simulink model "EPA_Jumper"  (R2018a)
settings: Solver=FixedStepDiscrete  StartTime=0.0  StopTime=inf  FixedStep=0.001  RelTol=1e-3  EnableMultiTasking=on
model workspace (MAT data in the model file):
  k_p_pam = Simulink.Parameter
  k_p_pam.DataType = 'auto'
  k_p_pam.Dimensions = [0 0]
values from neighbouring files (symbols this model uses):
  bits_current = 12    [Init_EPA_Jumper.m]
  bits_Kd = 12    [Init_EPA_Jumper.m]
  bits_Kp = 12    [Init_EPA_Jumper.m]
  bits_position = 16    [Init_EPA_Jumper.m]
  bits_velocity = 12    [Init_EPA_Jumper.m]
  KD_MAX = 5.0    (= 5)    [Init_EPA_Jumper.m]
  KD_MIN = 0.0    (= 0)    [Init_EPA_Jumper.m]
  KP_MAX = 500.0    (= 500)    [Init_EPA_Jumper.m]
  KP_MIN = 0.0    (= 0)    [Init_EPA_Jumper.m]
  P_MAX = 95.5    [Init_EPA_Jumper.m]
  P_MIN = -95.5    [Init_EPA_Jumper.m]
  PressureFilter_CutOffFreq = 20    [Init_EPA_Jumper.m]
  PressureFilter_Gain = 1    [Init_EPA_Jumper.m]
  ReadingVoltage = 5    [Init_EPA_Jumper.m]
  T_MAX = 18.0    (= 18)    [Init_EPA_Jumper.m]
  T_MIN = -18.0    (= -18)    [Init_EPA_Jumper.m]
  V_MAX = 45.0    (= 45)    [Init_EPA_Jumper.m]
  V_MIN = -45.0    (= -45)    [Init_EPA_Jumper.m]
  voltageBias = -2.5    [Init_EPA_Jumper.m]
  voltageMultiplier = 2.5    [Init_EPA_Jumper.m]
  VoltageResolution = 1023.0    (= 1023)    [Init_EPA_Jumper.m]
libraries: xpcethercatlib x76, slrtlib x15, simulink x10, peGeneralControl x9
(part 1 of 3)
settings Model: xpc_rtwmakecfg_data=_xpcethercatlib_  SimulationMode=external  Creator=marcm  LastModifiedBy=Lauflabor
settings SolverCC: ConcurrentTasks=on  AutoInsertRateTranBlk=on
settings DataIOCC: SaveFormat=StructureWithTime
settings OptimizationCC: BlockReduction=off  OptimizeBlockIOStorage=off  BufferReuse=off  GlobalBufferReuse=off  ExpressionFolding=off  LocalBlockOutputs=off  OptimizeDataStoreBuffers=off  BusAssignmentInplaceUpdate=off
settings HardwareCC: ProdBitPerPointer=32  ProdBitPerSizeT=32  ProdBitPerPtrDiffT=32  ProdLargestAtomicFloat=None  ProdWordSize=32  ProdLongLongMode=on  ProdHWDeviceType=Generic->32-bit x86 compatible
settings RTWCC: SystemTargetFile=slrt.tlc  TemplateMakefile=slrt_default_tmf  Description=Simulink Real-Time  CodeExecutionProfiling=on  RTWCompilerOptimization=on
settings CodeAppCC: StateflowObjectComments=on
settings SimulinkRealTimeCC: SupportVariableSizeSignals=on  xPCConcurrentTasks=on

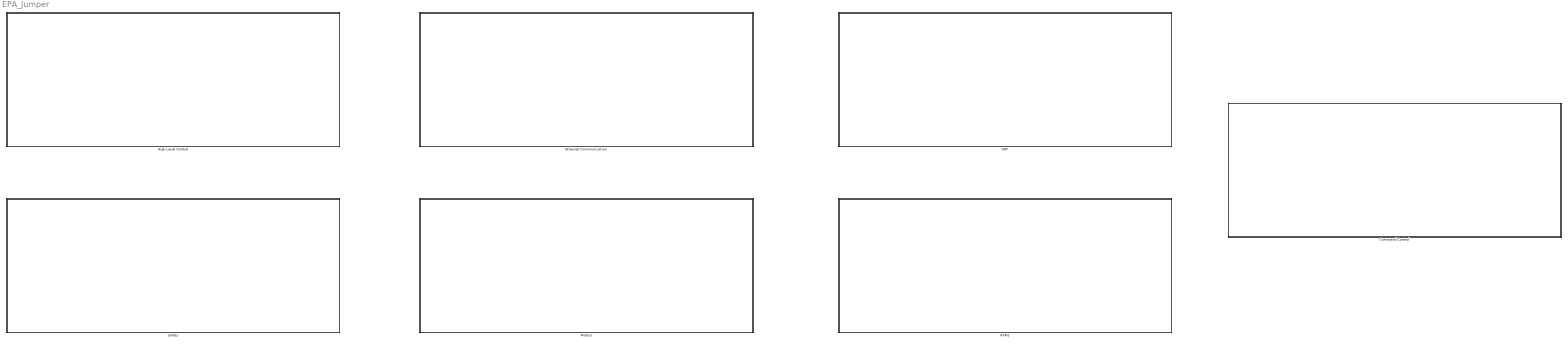
== system EPA_Jumper ==
  Command Control : Subsystem
  Ethernet Communication : Subsystem
  GRF : Subsystem
  High Level Control : Subsystem
  Motors : Subsystem
  PAMs : Subsystem
  "Safety " : Subsystem

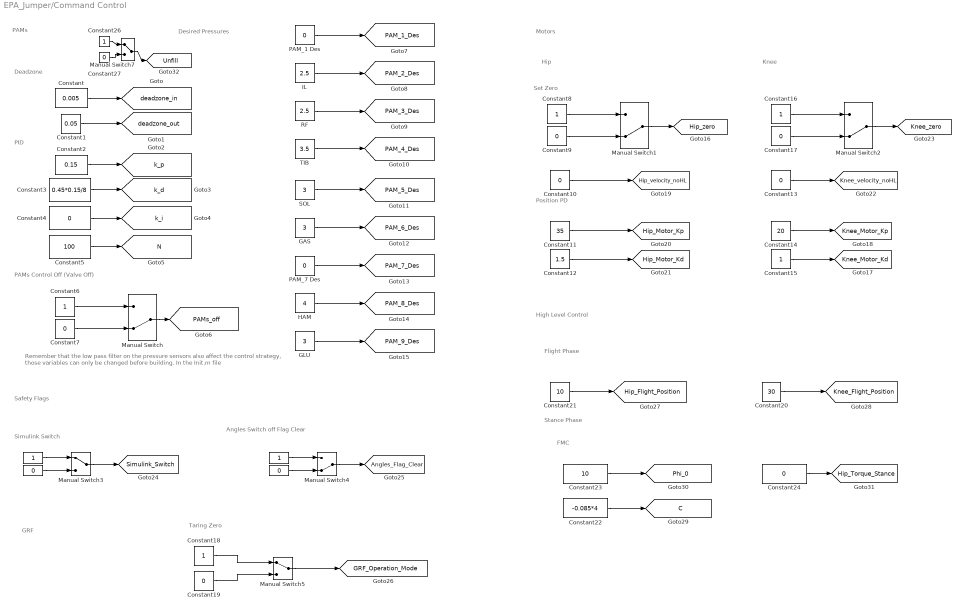
== system EPA_Jumper/Command Control ==
  note: PID
  note: PAMs
  note: Deadzone
  note: PAMs Control Off (Valve Off)
  note: Desired Pressures
  note: Motors
  note: Remember that the low pass filter on the pressure sensors also affect the control strategy, those variables can only be changed before building. In the Init.m file
  note: Hip
  note: Knee
  note: Safety Flags
  note: Simulink Switch
  note: Angles Switch off Flag Clear
  note: Taring Zero
  note: GRF
  note: High Level Control
  note: Flight Phase
  note: Stance Phase
  note: FMC
  note: Position PD
  note: Set Zero
  " " : Constant
  "   " : Constant  Value=0
  "    " : Constant  Value=0
  "               " : Constant
  Constant : Constant  Value=0.005
  Constant1 : Constant  Value=0.05
  Constant{4,7,9..10,13,17,19,24,27} (9 alike) : Constant  Value=0
  Constant11 : Constant  Value=35
  Constant12 : Constant  Value=1.5
  Constant14 : Constant  Value=20
  Constant{6,8,15..16,18,26} (6 alike) : Constant
  Constant2 : Constant  Value=0.15
  Constant20 : Constant  Value=30
  Constant21 : Constant  Value=10
  Constant22 : Constant  Value=-0.085*4
  Constant23 : Constant  Value=10
  Constant3 : Constant  Value=0.45*0.15/8
  Constant5 : Constant  Value=100
  GAS : Constant  Value=3
  GLU : Constant  Value=3
  HAM : Constant  Value=4
  IL : Constant  Value=2.5
  Manual Switch{,1..2,4} (4 alike) : ManualSwitch  CurrentSetting=0
  Manual Switch3 : ManualSwitch
  Manual Switch5 : ManualSwitch
  Manual Switch7 : ManualSwitch
  PAM_1 Des : Constant  Value=0
  PAM_7 Des : Constant  Value=0
  RF : Constant  Value=2.5
  SOL : Constant  Value=3
  TIB : Constant  Value=3.5
  tag scope: Angles_Flag_Clear=global, C=global, GRF_Operation_Mode=global, Hip_Flight_Position=global, Hip_Motor_Kd=global, Hip_Motor_Kp=global, Hip_Torque_Stance=global, Hip_velocity_noHL=global, Hip_zero=global, Knee_Flight_Position=global, Knee_Motor_Kd=global, Knee_Motor_Kp=global, Knee_velocity_noHL=global, Knee_zero=global, N=global, PAM_1_Des=global, PAM_2_Des=global, PAM_3_Des=global, PAM_4_Des=global, PAM_5_Des=global, PAM_6_Des=global, PAM_7_Des=global, PAM_8_Des=global, PAM_9_Des=global, PAMs_off=global, Phi_0=global, Simulink_Switch=global, Unfill=global, deadzone_in=global, deadzone_out=global, k_d=global, k_i=global, k_p=global
  wires:
  Constant5/1 -> [N]
  Constant4/1 -> [k_i]
  Constant6/1 -> Manual Switch/1
  Manual Switch/1 -> [PAMs_off]
  Constant1/1 -> [deadzone_out]
  Constant7/1 -> Manual Switch/2
  Constant2/1 -> [k_p]
  Constant/1 -> [deadzone_in]
  Constant3/1 -> [k_d]
  PAM_1 Des/1 -> [PAM_1_Des]
  IL/1 -> [PAM_2_Des]
  RF/1 -> [PAM_3_Des]
  TIB/1 -> [PAM_4_Des]
  SOL/1 -> [PAM_5_Des]
  GAS/1 -> [PAM_6_Des]
  PAM_7 Des/1 -> [PAM_7_Des]
  HAM/1 -> [PAM_8_Des]
  GLU/1 -> [PAM_9_Des]
  Constant8/1 -> Manual Switch1/1
  Constant9/1 -> Manual Switch1/2
  Manual Switch1/1 -> [Hip_zero]
  Constant10/1 -> [Hip_velocity_noHL]
  Constant11/1 -> [Hip_Motor_Kp]
  Constant12/1 -> [Hip_Motor_Kd]
  Constant13/1 -> [Knee_velocity_noHL]
  Constant14/1 -> [Knee_Motor_Kp]
  Constant15/1 -> [Knee_Motor_Kd]
  Manual Switch2/1 -> [Knee_zero]
  Constant17/1 -> Manual Switch2/2
  Constant16/1 -> Manual Switch2/1
  " "/1 -> Manual Switch3/1
  "    "/1 -> Manual Switch3/2
  Manual Switch3/1 -> [Simulink_Switch]
  Manual Switch4/1 -> [Angles_Flag_Clear]
  "               "/1 -> Manual Switch4/1
  "   "/1 -> Manual Switch4/2
  Manual Switch5/1 -> [GRF_Operation_Mode]
  Constant18/1 -> Manual Switch5/1
  Constant19/1 -> Manual Switch5/2
  Constant21/1 -> [Hip_Flight_Position]
  Constant20/1 -> [Knee_Flight_Position]
  Constant23/1 -> [Phi_0]
  Constant22/1 -> [C]
  Constant24/1 -> [Hip_Torque_Stance]
  Constant26/1 -> Manual Switch7/1
  Constant27/1 -> Manual Switch7/2
  Manual Switch7/1 -> [Unfill]

== system EPA_Jumper/Ethernet Communication ==
  "EtherCAT Get Notifications " : xpcethercatlib/EtherCAT Get Notifications   device_id=0  sample_time=.001
      settings: SourceProductName=Simulink Real-Time  SourceProductBaseCode=XP
  "EtherCAT Init " : xpcethercatlib/EtherCAT Init   Priority=0  config_file=C:\Users\Lauflabor\Documents\EPA Jumper\RealTime Code\EPA_Jumper_2.xml  device_id=0  pci_bus=1  pci_slot=0  pci_function=0  dctuning=0  enaDebug=on  enaDC=on  errLink=off  masterDbg=on  stateChgDbg=on  baseClock=on  masterCfg=off  logFile='c:\dbglog.txt'  sample_time=0.001000  DCMode=0
      settings: SourceProductName=Simulink Real-Time  SourceProductBaseCode=XP
  Inputs : Subsystem
  Outputs : Subsystem
  Terminator : Terminator
  Terminator1 : Terminator
  wires:
  "EtherCAT Get Notifications "/1 -> Terminator1/1
  "EtherCAT Init "/1 -> Terminator/1

== system EPA_Jumper/GRF ==
  note: GRF Meassures
  GRFx : Subsystem
  GRFy : Subsystem
  GRFz : Subsystem

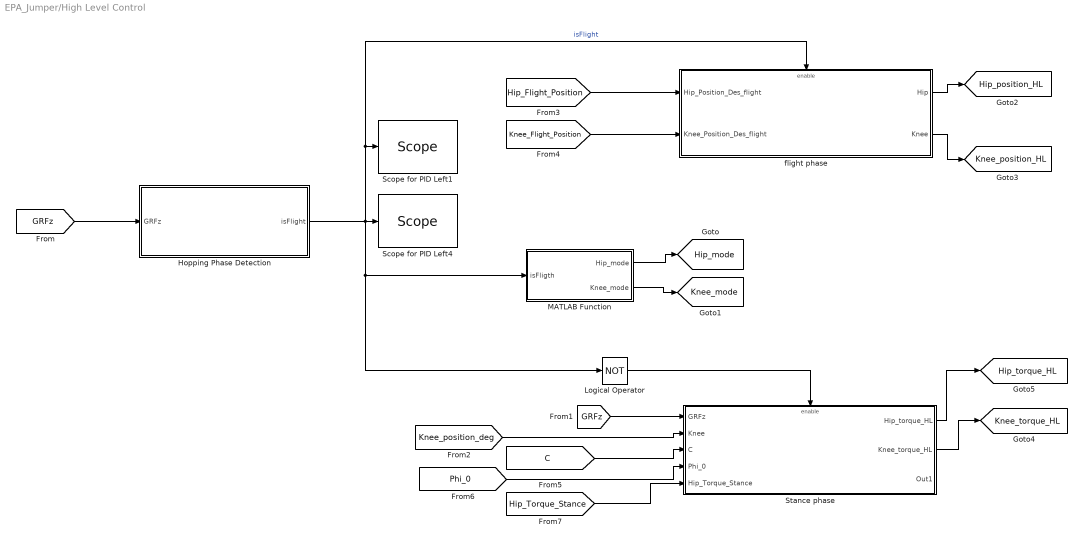
== system EPA_Jumper/High Level Control ==
  Hopping Phase Detection : MATLAB Function  TreatAsAtomicUnit=on
  Logical Operator : Logic  Operator=NOT  AllPortsSameDT=off  OutDataTypeStr=boolean
  MATLAB Function : MATLAB Function  TreatAsAtomicUnit=on
  Scope for PID Left1 : slrtlib/Displays and Logging/Scope   scopeno=7  scopetype=File  autostart=on  viewmode=Graphical sliding  formatstr='%15.6f'  grid=on  ylimits=[-0.5, 1.5]  nosamples=1000000  noprepostsamples=0  interleave=1  triggermode=FreeRun  triggersignal=1  trigsignalfromport=off  triggerlevel=0.0  triggerslope=Either  triggerscope=1  triggersample=0  filename=isFlight.dat  mode=Lazy  writesize=512  autorestart=off  dynamicfilemode=off  maxwritefilesize=512*1024^2
  Scope for PID Left4 : slrtlib/Displays and Logging/Scope   scopeno=6  scopetype=Target  autostart=on  viewmode=Graphical sliding  formatstr='%15.6f'  grid=on  ylimits=[-0.5, 1.5]  nosamples=1000  noprepostsamples=0  interleave=1  triggermode=FreeRun  triggersignal=1  trigsignalfromport=off  triggerlevel=0.0  triggerslope=Either  triggerscope=1  triggersample=0  filename=data.dat  mode=Lazy  writesize=512  autorestart=off  dynamicfilemode=off  maxwritefilesize=512*1024^2
  Stance phase : Subsystem
  flight phase : Subsystem
  tag scope: Hip_mode=global, Hip_position_HL=global, Hip_torque_HL=global, Knee_mode=global, Knee_position_HL=global, Knee_torque_HL=global
  wires:
  Hopping Phase Detection/1(isFlight) -> Scope for PID Left1/1, flight phase/Enable, Scope for PID Left4/1, MATLAB Function/1(isFligth), Logical Operator/1  "isFlight"
  [GRFz] -> Hopping Phase Detection/1(GRFz)
  [Hip_Flight_Position] -> flight phase/1(Hip_Position_Des_flight)
  [Knee_Flight_Position] -> flight phase/2(Knee_Position_Des_flight)
  Logical Operator/1 -> Stance phase/Enable
  MATLAB Function/1(Hip_mode) -> [Hip_mode]
  MATLAB Function/2(Knee_mode) -> [Knee_mode]
  flight phase/1(Hip) -> [Hip_position_HL]
  flight phase/2(Knee) -> [Knee_position_HL]
  [GRFz] -> Stance phase/1("GRFz ")
  [Knee_position_deg] -> Stance phase/2(Knee)
  Stance phase/2(Knee_torque_HL) -> [Knee_torque_HL]
  Stance phase/1(Hip_torque_HL) -> [Hip_torque_HL]
  [C] -> Stance phase/3(C)
  [Phi_0] -> Stance phase/4(Phi_0)
  [Hip_Torque_Stance] -> Stance phase/5(Hip_Torque_Stance)

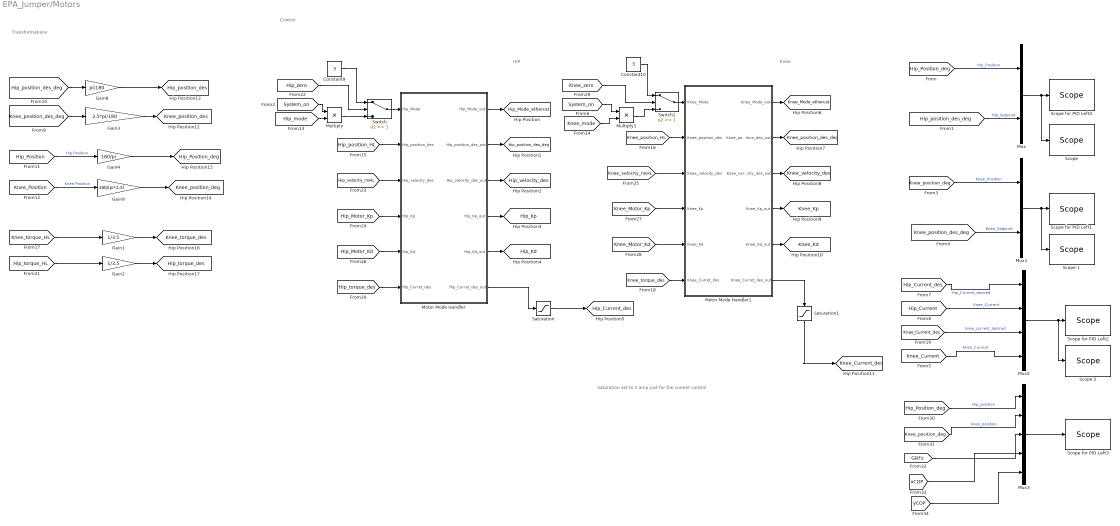
== system EPA_Jumper/Motors ==
  note: Saturation set to 5 amp just for the current control
  note: HIP
  note: Knee
  note: Control
  note: Transformations
  Constant10 : Constant  Value=3
  Constant9 : Constant  Value=3
  Gain1 : Gain  Gain=1/3.5
  Gain2 : Gain  Gain=1/3.5
  Gain3 : Gain  Gain=2.5*pi/180
  Gain4 : Gain  Gain=180/pi
  Gain8 : Gain  Gain=pi/180
  Gain9 : Gain  Gain=180/(pi*2.5)
  Motor Mode Handler : MATLAB Function  TreatAsAtomicUnit=on
  Motor Mode Handler1 : MATLAB Function  TreatAsAtomicUnit=on
  Multiply : Product
  Multiply1 : Product
  Mux : Mux  Inputs=2
  Mux1 : Mux  Inputs=2
  Mux2 : Mux
  Mux3 : Mux  Inputs=5
  Saturation : Saturate  UpperLimit=10  LowerLimit=-10
  Saturation1 : Saturate  UpperLimit=10  LowerLimit=-10
  "Scope " : slrtlib/Displays and Logging/Scope   scopeno=12  scopetype=File  autostart=on  viewmode=Graphical redraw  formatstr='%15.6f'  grid=on  ylimits=[0,0]  nosamples=1000000  noprepostsamples=0  interleave=1  triggermode=FreeRun  triggersignal=1  trigsignalfromport=off  triggerlevel=0.0  triggerslope=Either  triggerscope=1  triggersample=0  filename=hipPos.dat  mode=Lazy  writesize=512  autorestart=off  dynamicfilemode=off  maxwritefilesize=512*1024^2
  Scope 1 : slrtlib/Displays and Logging/Scope   scopeno=13  scopetype=File  autostart=on  viewmode=Graphical redraw  formatstr='%15.6f'  grid=on  ylimits=[0,0]  nosamples=1000000  noprepostsamples=0  interleave=1  triggermode=FreeRun  triggersignal=1  trigsignalfromport=off  triggerlevel=0.0  triggerslope=Either  triggerscope=1  triggersample=0  filename=kneePos.dat  mode=Lazy  writesize=512  autorestart=off  dynamicfilemode=off  maxwritefilesize=512*1024^2
  Scope 2 : slrtlib/Displays and Logging/Scope   scopeno=14  scopetype=File  autostart=on  viewmode=Graphical redraw  formatstr='%15.6f'  grid=on  ylimits=[0,0]  nosamples=1000000  noprepostsamples=0  interleave=1  triggermode=FreeRun  triggersignal=1  trigsignalfromport=off  triggerlevel=0.0  triggerslope=Either  triggerscope=1  triggersample=0  filename=motCurr.dat  mode=Lazy  writesize=512  autorestart=off  dynamicfilemode=off  maxwritefilesize=512*1024^2
  Scope for PID Left1 : slrtlib/Displays and Logging/Scope   scopeno=4  scopetype=Target  autostart=on  viewmode=Graphical sliding  formatstr='%15.6f'  grid=on  ylimits=[-10, 120]  nosamples=1000  noprepostsamples=0  interleave=1  triggermode=FreeRun  triggersignal=1  trigsignalfromport=off  triggerlevel=0.0  triggerslope=Either  triggerscope=1  triggersample=0  filename=data.dat  mode=Lazy  writesize=512  autorestart=off  dynamicfilemode=off  maxwritefilesize=512*1024^2
  Scope for PID Left2 : slrtlib/Displays and Logging/Scope   scopeno=5  scopetype=Target  autostart=on  viewmode=Numerical  formatstr='%15.6f'  grid=on  ylimits=[0, 0]  nosamples=1000  noprepostsamples=0  interleave=1  triggermode=FreeRun  triggersignal=1  trigsignalfromport=off  triggerlevel=0.0  triggerslope=Either  triggerscope=1  triggersample=0  filename=data.dat  mode=Lazy  writesize=512  autorestart=off  dynamicfilemode=off  maxwritefilesize=512*1024^2
  Scope for PID Left3 : slrtlib/Displays and Logging/Scope   scopeno=9  scopetype=Target  autostart=on  viewmode=Numerical  formatstr='%15.6f'  grid=on  ylimits=[0, 0]  nosamples=500  noprepostsamples=0  interleave=1  triggermode=FreeRun  triggersignal=1  trigsignalfromport=off  triggerlevel=0.0  triggerslope=Either  triggerscope=1  triggersample=0  filename=data.dat  mode=Lazy  writesize=512  autorestart=off  dynamicfilemode=off  maxwritefilesize=512*1024^2
  Scope for PID Left4 : slrtlib/Displays and Logging/Scope   scopeno=3  scopetype=Target  autostart=on  viewmode=Graphical sliding  formatstr='%15.6f'  grid=on  ylimits=[-60, 60]  nosamples=1000  noprepostsamples=0  interleave=1  triggermode=FreeRun  triggersignal=1  trigsignalfromport=off  triggerlevel=0.0  triggerslope=Either  triggerscope=1  triggersample=0  filename=data.dat  mode=Lazy  writesize=512  autorestart=off  dynamicfilemode=off  maxwritefilesize=512*1024^2
  Switch : Switch  Threshold=1
  Switch1 : Switch  Threshold=1
  tag scope: Hip_Current_des=global, Hip_Kd=global, Hip_Kp=global, Hip_Mode_ethercat=global, Hip_Position_deg=global, Hip_position_des=global, Hip_position_des_deg=global, Hip_torque_des=global, Hip_velocity_des=global, Knee_Current_des=global, Knee_Kd=global, Knee_Kp=global, Knee_Mode_ethercat=global, Knee_position_deg=global, Knee_position_des=global, Knee_position_des_deg=global, Knee_torque_des=global, Knee_velocity_des=global
  wires:
  Motor Mode Handler/3(Hip_velocity_des_out) -> [Hip_velocity_des]
  Motor Mode Handler/4(Hip_Kp_out) -> [Hip_Kp]
  Motor Mode Handler/5(Hip_Kd_out) -> [Hip_Kd]
  Motor Mode Handler/6(Hip_Curret_des_out) -> Saturation/1
  Motor Mode Handler/2(Hip_position_des_out) -> [Hip_position_des_deg]
  [Hip_position_des_deg] -> Mux/2  "Hip_Setpoint"
  [Hip_Position_deg] -> Mux/1  "Hip_Position"
  Mux/1 -> "Scope "/1, Scope for PID Left4/1
  Mux1/1 -> Scope 1/1, Scope for PID Left1/1
  [Knee_position_des_deg] -> Mux1/2  "Knee_Setpoint"
  Mux2/1 -> Scope 2/1, Scope for PID Left2/1
  Multiply/1 -> Switch/3
  [System_on] -> Multiply/1
  Motor Mode Handler/1(Hip_Mode_out) -> [Hip_Mode_ethercat]
  [Hip_position_HL] -> Motor Mode Handler/2(Hip_position_des)
  [Hip_velocity_noHL] -> Motor Mode Handler/3(Hip_velocity_des)
  [Hip_Motor_Kp] -> Motor Mode Handler/4(Hip_Kp)
  [Hip_Motor_Kd] -> Motor Mode Handler/5(Hip_Kd)
  [Hip_torque_des] -> Motor Mode Handler/6(Hip_Curret_des)
  [Knee_position_HL] -> Motor Mode Handler1/2(Knee_position_des)
  [System_on] -> Multiply1/1
  Motor Mode Handler1/5(Knee_Kd_out) -> [Knee_Kd]
  Motor Mode Handler1/1(Knee_Mode_out) -> [Knee_Mode_ethercat]
  Motor Mode Handler1/2(Knee_position_des_out) -> [Knee_position_des_deg]
  Motor Mode Handler1/3(Knee_velocity_des_out) -> [Knee_velocity_des]
  Motor Mode Handler1/4(Knee_Kp_out) -> [Knee_Kp]
  Motor Mode Handler1/6(Knee_Curret_des_out) -> Saturation1/1
  [Knee_position_deg] -> Mux1/1  "Knee_Position"
  [Hip_position_des_deg] -> Gain8/1
  [Knee_position_des_deg] -> Gain3/1
  [Hip_Position] -> Gain4/1  "Hip Position"
  [Knee_Position] -> Gain9/1  "Knee Position"
  Gain3/1 -> [Knee_position_des]
  Gain8/1 -> [Hip_position_des]
  Gain9/1 -> [Knee_position_deg]
  Gain4/1 -> [Hip_Position_deg]
  [Knee_torque_HL] -> Gain1/1
  Gain1/1 -> [Knee_torque_des]
  [Hip_mode] -> Multiply/2
  Constant9/1 -> Switch/1
  [Knee_mode] -> Multiply1/2
  Constant10/1 -> Switch1/1
  Switch/1 -> Motor Mode Handler/1(Hip_Mode)
  Switch1/1 -> Motor Mode Handler1/1(Knee_Mode)
  [Knee_torque_des] -> Motor Mode Handler1/6(Knee_Curret_des)
  Saturation/1 -> [Hip_Current_des]
  Saturation1/1 -> [Knee_Current_des]
  [Hip_torque_HL] -> Gain2/1
  Gain2/1 -> [Hip_torque_des]
  [Hip_zero] -> Switch/2
  [Knee_velocity_noHL] -> Motor Mode Handler1/3(Knee_velocity_des)
  [Knee_Motor_Kp] -> Motor Mode Handler1/4(Knee_Kp)
  [Knee_Motor_Kd] -> Motor Mode Handler1/5(Knee_Kd)
  Multiply1/1 -> Switch1/3
  [Knee_zero] -> Switch1/2
  Mux3/1 -> Scope for PID Left3/1
  [Hip_Position_deg] -> Mux3/1  "Hip_position"
  [Knee_position_deg] -> Mux3/2  "knee_position"
  [Hip_Current_des] -> Mux2/1  "Hip_Current_desired"
  [Hip_Current] -> Mux2/2  "Knee_Current"
  [Knee_Current_des] -> Mux2/3  "knee_current_desired"
  [Knee_Current] -> Mux2/4  "Knee_Current"
  [GRFz] -> Mux3/3
  [xCOP] -> Mux3/4
  [yCOP] -> Mux3/5

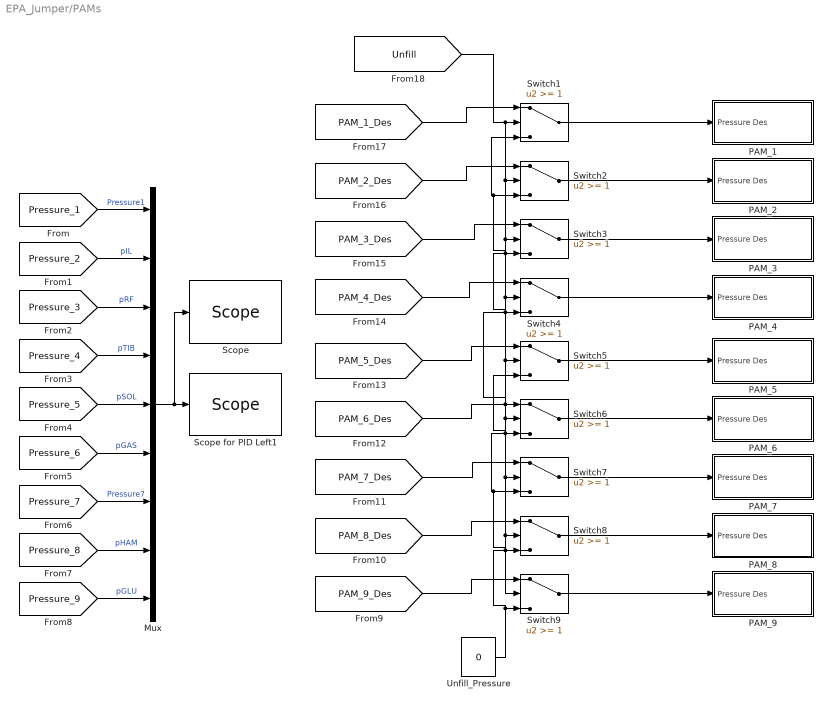
== system EPA_Jumper/PAMs ==
  Mux : Mux  Inputs=9
  PAM_1 : Subsystem
  PAM_2 : Subsystem
  PAM_3 : Subsystem
  PAM_4 : Subsystem
  PAM_5 : Subsystem
  PAM_6 : Subsystem
  PAM_7 : Subsystem
  PAM_8 : Subsystem
  PAM_9 : Subsystem
  "Scope " : slrtlib/Displays and Logging/Scope   scopeno=15  scopetype=File  autostart=on  viewmode=Graphical redraw  formatstr='%15.6f'  grid=on  ylimits=[0,0]  nosamples=1000000  noprepostsamples=0  interleave=1  triggermode=FreeRun  triggersignal=1  trigsignalfromport=off  triggerlevel=0.0  triggerslope=Either  triggerscope=1  triggersample=0  filename=pressure.dat  mode=Lazy  writesize=512  autorestart=off  dynamicfilemode=off  maxwritefilesize=512*1024^2
  Scope for PID Left1 : slrtlib/Displays and Logging/Scope   scopeno=8  scopetype=Target  autostart=on  viewmode=Numerical  formatstr='%15.6f'  grid=on  ylimits=[0, 120]  nosamples=1000  noprepostsamples=0  interleave=1  triggermode=FreeRun  triggersignal=1  trigsignalfromport=off  triggerlevel=0.0  triggerslope=Either  triggerscope=1  triggersample=0  filename=data.dat  mode=Lazy  writesize=512  autorestart=off  dynamicfilemode=off  maxwritefilesize=512*1024^2
  Switch{1..9} (9 alike) : Switch  Threshold=1
  Unfill_Pressure : Constant  Value=0
  wires:
  Mux/1 -> "Scope "/1, Scope for PID Left1/1
  [Pressure_1] -> Mux/1  "Pressure1"
  [Pressure_2] -> Mux/2  "pIL"
  [Pressure_3] -> Mux/3  "pRF"
  [Pressure_4] -> Mux/4  "pTIB"
  [Pressure_5] -> Mux/5  "pSOL"
  [Pressure_6] -> Mux/6  "pGAS"
  [Pressure_7] -> Mux/7  "Pressure7"
  [Pressure_8] -> Mux/8  "pHAM"
  [Pressure_9] -> Mux/9  "pGLU"
  [PAM_9_Des] -> Switch9/1
  Switch8/1 -> PAM_8/1(Pressure Des)
  Switch7/1 -> PAM_7/1(Pressure Des)
  [PAM_7_Des] -> Switch7/1
  [PAM_8_Des] -> Switch8/1
  [PAM_1_Des] -> Switch1/1
  Switch1/1 -> PAM_1/1(Pressure Des)
  [PAM_2_Des] -> Switch2/1
  Switch2/1 -> PAM_2/1(Pressure Des)
  [PAM_3_Des] -> Switch3/1
  Switch3/1 -> PAM_3/1(Pressure Des)
  [PAM_4_Des] -> Switch4/1
  Switch4/1 -> PAM_4/1(Pressure Des)
  [PAM_5_Des] -> Switch5/1
  Switch5/1 -> PAM_5/1(Pressure Des)
  Switch6/1 -> PAM_6/1(Pressure Des)
  [PAM_6_Des] -> Switch2/3, Switch1/3, Switch3/3, Switch4/3, Switch6/1
  [Unfill] -> Switch9/2, Switch8/2, Switch7/2, Switch6/2, Switch5/2, Switch4/2, Switch3/2, Switch2/2, Switch1/2
  Switch9/1 -> PAM_9/1(Pressure Des)
  Unfill_Pressure/1 -> Switch7/3, Switch5/3, Switch6/3, Switch8/3, Switch9/3

== system EPA_Jumper/Safety  ==
  AND1 : Logic  IconShape=distinctive  AllPortsSameDT=off  OutDataTypeStr=boolean
  Delay : Delay  DelayLength=1  InitialCondition=0  ExternalReset=Either
      settings: InputPortMap=u0,r5
  MATLAB Function : MATLAB Function  TreatAsAtomicUnit=on
  Mux : Mux  Inputs=6
  "Scope " : slrtlib/Displays and Logging/Scope   scopeno=11  scopetype=File  autostart=on  viewmode=Graphical redraw  formatstr='%15.6f'  grid=on  ylimits=[0,0]  nosamples=1000000  noprepostsamples=0  interleave=1  triggermode=FreeRun  triggersignal=1  trigsignalfromport=off  triggerlevel=0.0  triggerslope=Either  triggerscope=1  triggersample=0  filename=safety.dat  mode=Lazy  writesize=512  autorestart=off  dynamicfilemode=off  maxwritefilesize=512*1024^2
  Scope for PID Left4 : slrtlib/Displays and Logging/Scope   scopeno=2  scopetype=Target  autostart=on  viewmode=Numerical  formatstr='%15.6f'  grid=on  ylimits=[0, 0]  nosamples=1000  noprepostsamples=0  interleave=1  triggermode=FreeRun  triggersignal=1  trigsignalfromport=off  triggerlevel=0.0  triggerslope=Either  triggerscope=1  triggersample=0  filename=data.dat  mode=Lazy  writesize=512  autorestart=off  dynamicfilemode=off  maxwritefilesize=512*1024^2
  System On : Subsystem
  tag scope: System_on=global
  wires:
  System On/1(System On) -> Mux/1, AND1/1  "System_On"
  [Simulink_Switch] -> Mux/2, System On/1("Simulink Switch ")  "Simulink_wwitch"
  Mux/1 -> "Scope "/1, Scope for PID Left4/1
  System On/2(Emergency) -> Mux/3  "Emergency_switch"
  [Hip_Position_deg] -> MATLAB Function/1(Hip_Position)
  [Knee_position_deg] -> MATLAB Function/2(Knee_Position)
  MATLAB Function/3(Motors_safe) -> AND1/2, Mux/4  "Motors_safe"
  MATLAB Function/1(Hip_motor_safe) -> Mux/5  "Hip_motor_safe"
  MATLAB Function/2(Knee_motor_safe) -> Mux/6  "Knee_motor_safe"
  AND1/1 -> [System_on]  "System_On"
  MATLAB Function/4(flag) -> Delay/1
  Delay/1 -> MATLAB Function/3(flag_1)
  [Angles_Flag_Clear] -> Delay/2

== system EPA_Jumper/Ethernet Communication/Inputs ==
  GRF Slave : Subsystem
  Motor Slave : Subsystem
  PAMs Slave : Subsystem

== system EPA_Jumper/Ethernet Communication/Outputs ==
  GRF Slave : Subsystem
  Motor Slave : Subsystem
  PAMs Slave : Subsystem

== system EPA_Jumper/GRF/GRFx ==

== system EPA_Jumper/GRF/GRFy ==

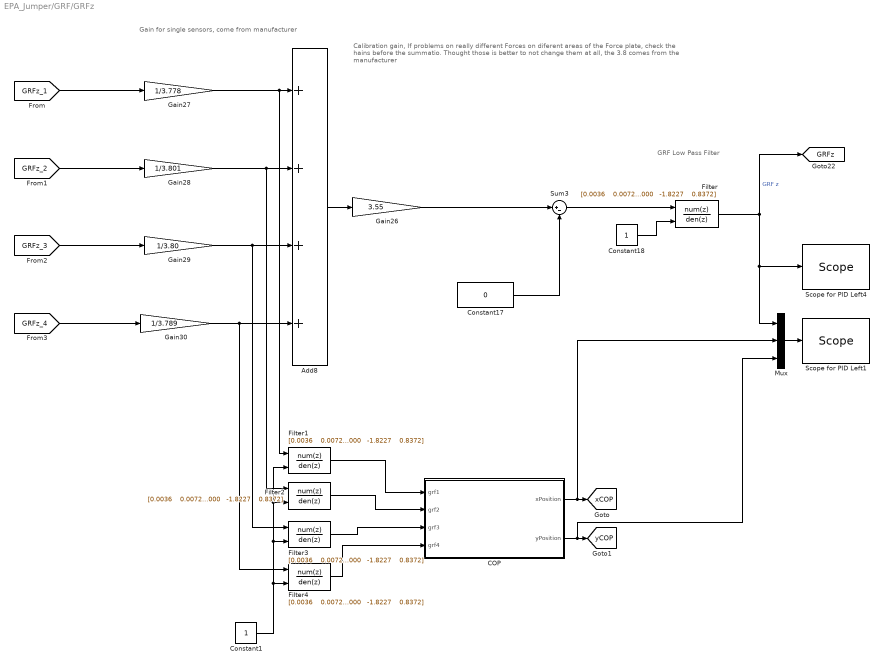
== system EPA_Jumper/GRF/GRFz ==
  note: Calibration gain, If problems on really different Forces on diferent areas of the Force plate, check the hains before the summatio. Thought those is better to not change them at all, the 3.8 comes from the manufacturer
  note: GRF Low Pass Filter
  note: Gain for single sensors, come from manufacturer
  Add8 : Sum  Inputs=++++
  COP : MATLAB Function  TreatAsAtomicUnit=on
  Constant1 : Constant
  Constant17 : Constant  Value=0
  Constant18 : Constant
  Filter{,1..4} (5 alike) : DiscreteFilter  Numerator="[0.0036    0.0072    0.0036]"  Denominator="[1.0000   -1.8227    0.8372]"  ExternalReset=Either
      settings: InputPortMap=u0,r7
  Gain26 : Gain  Gain=3.55
  Gain27 : Gain  Gain=1/3.778
  Gain28 : Gain  Gain=1/3.801
  Gain29 : Gain  Gain=1/3.80
  Gain30 : Gain  Gain=1/3.789
  Mux : Mux  Inputs=3
  Scope for PID Left1 : slrtlib/Displays and Logging/Scope   scopeno=10  scopetype=File  autostart=on  viewmode=Graphical sliding  formatstr='%15.6f'  grid=on  ylimits=[0, 100]  nosamples=1000000  noprepostsamples=0  interleave=1  triggermode=FreeRun  triggersignal=1  trigsignalfromport=off  triggerlevel=0.0  triggerslope=Either  triggerscope=1  triggersample=0  filename=grf.dat  mode=Lazy  writesize=512  autorestart=off  dynamicfilemode=off  maxwritefilesize=512*1024^2
  Scope for PID Left4 : slrtlib/Displays and Logging/Scope   scopeno=1  scopetype=Target  autostart=on  viewmode=Graphical sliding  formatstr='%15.6f'  grid=on  ylimits=[0, 100]  nosamples=1000  noprepostsamples=0  interleave=1  triggermode=FreeRun  triggersignal=1  trigsignalfromport=off  triggerlevel=0.0  triggerslope=Either  triggerscope=1  triggersample=0  filename=data.dat  mode=Lazy  writesize=512  autorestart=off  dynamicfilemode=off  maxwritefilesize=512*1024^2
  Sum3 : Sum  Inputs=|+-
  tag scope: GRFz=global, xCOP=global, yCOP=global
  wires:
  Gain26/1 -> Sum3/1
  Constant18/1 -> Filter/2
  Constant17/1 -> Sum3/2
  Sum3/1 -> Filter/1
  Gain29/1 -> Add8/3, Filter3/1
  [GRFz_3] -> Gain29/1
  Gain28/1 -> Filter2/1, Add8/2
  [GRFz_1] -> Gain27/1
  Filter/1 -> [GRFz], Mux/1, Scope for PID Left4/1  "GRF z"
  [GRFz_4] -> Gain30/1
  [GRFz_2] -> Gain28/1
  Gain30/1 -> Filter4/1, Add8/4
  Gain27/1 -> Filter1/1, Add8/1
  Add8/1 -> Gain26/1
  Constant1/1 -> Filter2/2, Filter1/2, Filter3/2, Filter4/2
  Filter1/1 -> COP/1(grf1)
  Filter2/1 -> COP/2(grf2)
  Filter3/1 -> COP/3(grf3)
  Filter4/1 -> COP/4(grf4)
  COP/2(yPosition) -> Mux/3, [yCOP]
  COP/1(xPosition) -> Mux/2, [xCOP]
  Mux/1 -> Scope for PID Left1/1

== system EPA_Jumper/High Level Control/Stance phase ==
  "GRFz " : Inport
  Knee : Inport  Port=2
  C : Inport  Port=3
  Phi_0 : Inport  Port=4
  Hip_Torque_Stance : Inport  Port=5
  Enable : EnablePort  StatesWhenEnabling=reset
  FMCK (Static) : Subsystem
  Mux : Mux  Inputs=2
  Hip_torque_HL : Outport
  Knee_torque_HL : Outport  Port=2
  Out1 : Outport  Port=3
  wires:
  "GRFz "/1 -> FMCK (Static)/1(GRF_Z)
  Knee/1 -> FMCK (Static)/2(angKne)
  FMCK (Static)/2(Phi0) -> Mux/1
  Mux/1 -> Out1/1
  FMCK (Static)/3(C) -> Mux/2
  FMCK (Static)/1(torMotKne) -> Knee_torque_HL/1
  Hip_Torque_Stance/1 -> Hip_torque_HL/1
  C/1 -> FMCK (Static)/3(C_)
  Phi_0/1 -> FMCK (Static)/4(Phi_0)

== system EPA_Jumper/High Level Control/flight phase ==
  Hip_Position_Des_flight : Inport
  Knee_Position_Des_flight : Inport  Port=2
  Enable : EnablePort  StatesWhenEnabling=reset
  Hip : Outport
  Knee : Outport  Port=2
  wires:
  Hip_Position_Des_flight/1 -> Hip/1
  Knee_Position_Des_flight/1 -> Knee/1

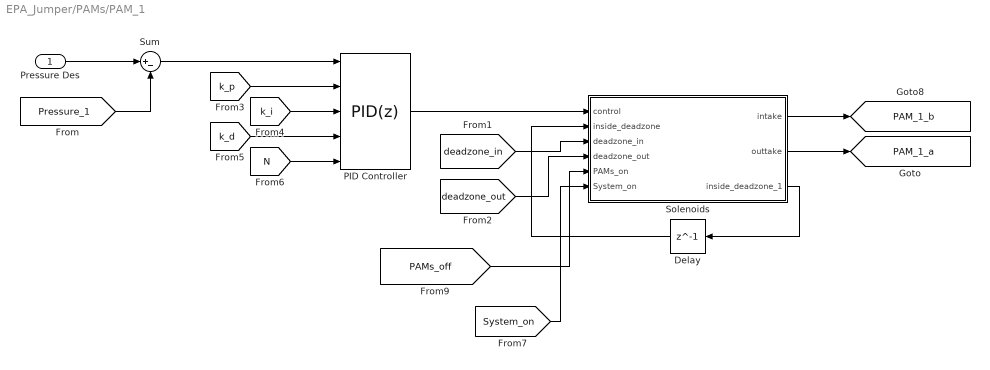
== system EPA_Jumper/PAMs/PAM_1 ==
  Pressure Des : Inport
  Delay : Delay  DelayLength=1
  PID Controller : simulink/Continuous/PID Controller  Controller=PID  TimeDomain=Discrete-time  SampleTime=-1  IntegratorMethod=Forward Euler  FilterMethod=Forward Euler  Form=Ideal  UseFilter=on  ControllerParametersSource=external  P=k_p_pam  I=0  D=0.45*0.15/8  N=100  InitialConditionSource=internal  InitialConditionForIntegrator=0  InitialConditionForFilter=0  ExternalReset=none  LimitOutput=off  UpperSaturationLimit=inf  LowerSaturationLimit=-inf  LinearizeAsGain=on  AntiWindupMode=none  Kb=1  TrackingMode=off  Kt=1  PParamMin=[]  PParamMax=[]  IParamMin=[]  IParamMax=[]  DParamMin=[]  DParamMax=[]  NParamMin=[]  NParamMax=[]  KbParamMin=[]  KbParamMax=[]  KtParamMin=[]  KtParamMax=[]  POutMin=[]  POutMax=[]  IOutMin=[]  IOutMax=[]  DOutMin=[]  DOutMax=[]  NOutMin=[]  NOutMax=[]  KbOutMin=[]  KbOutMax=[]  KtOutMin=[]  KtOutMax=[]  IntegratorOutMin=[]  IntegratorOutMax=[]  FilterOutMin=[]  FilterOutMax=[]  SumOutMin=[]  SumOutMax=[]  SumI1OutMin=[]  SumI1OutMax=[]  SumI2OutMin=[]  SumI2OutMax=[]  SumI3OutMin=[]  SumI3OutMax=[]  SumDOutMin=[]  SumDOutMax=[]  SaturationOutMin=[]  SaturationOutMax=[]  IntegratorContinuousStateAttributes=''  IntegratorStateMustResolveToSignalObject=off  IntegratorRTWStateStorageClass=Auto  FilterContinuousStateAttributes=''  FilterStateMustResolveToSignalObject=off  FilterRTWStateStorageClass=Auto  DifferentiatorICPrevScaledInput=0  DifferentiatorOutMin=[]  DifferentiatorOutMax=[]  FilterDiffOutCoefMin=[]  FilterDiffOutCoefMax=[]  SumDenOutMin=[]  SumDenOutMax=[]  SumNumOutMin=[]  SumNumOutMax=[]  ReciprocalOutMin=[]  ReciprocalOutMax=[]  DivideOutMin=[]  DivideOutMax=[]  TunerSelectOption=Transfer Function Based (PID Tuner App)
  Solenoids : MATLAB Function  TreatAsAtomicUnit=on
  Sum : Sum  Inputs=|+-
  tag scope: PAM_1_a=global, PAM_1_b=global
  wires:
  Solenoids/3(inside_deadzone_1) -> Delay/1
  Delay/1 -> Solenoids/2(inside_deadzone)
  PID Controller/1 -> Solenoids/1(control)
  Pressure Des/1 -> Sum/1
  [Pressure_1] -> Sum/2
  Sum/1 -> PID Controller/1
  [deadzone_in] -> Solenoids/3(deadzone_in)
  [deadzone_out] -> Solenoids/4(deadzone_out)
  Solenoids/1(intake) -> [PAM_1_b]
  Solenoids/2(outtake) -> [PAM_1_a]
  [k_p] -> PID Controller/2
  [k_i] -> PID Controller/3
  [k_d] -> PID Controller/4
  [N] -> PID Controller/5
  [PAMs_off] -> Solenoids/5(PAMs_on)
  [System_on] -> Solenoids/6(System_on)

== system EPA_Jumper/PAMs/PAM_2 ==
  Pressure Des : Inport
  Delay : Delay  DelayLength=1
  PID Controller : simulink/Continuous/PID Controller  Controller=PID  TimeDomain=Discrete-time  SampleTime=-1  IntegratorMethod=Forward Euler  FilterMethod=Forward Euler  Form=Ideal  UseFilter=on  ControllerParametersSource=external  P=k_p_pam  I=0  D=0.45*0.15/8  N=100  InitialConditionSource=internal  InitialConditionForIntegrator=0  InitialConditionForFilter=0  ExternalReset=none  LimitOutput=off  UpperSaturationLimit=inf  LowerSaturationLimit=-inf  LinearizeAsGain=on  AntiWindupMode=none  Kb=1  TrackingMode=off  Kt=1  PParamMin=[]  PParamMax=[]  IParamMin=[]  IParamMax=[]  DParamMin=[]  DParamMax=[]  NParamMin=[]  NParamMax=[]  KbParamMin=[]  KbParamMax=[]  KtParamMin=[]  KtParamMax=[]  POutMin=[]  POutMax=[]  IOutMin=[]  IOutMax=[]  DOutMin=[]  DOutMax=[]  NOutMin=[]  NOutMax=[]  KbOutMin=[]  KbOutMax=[]  KtOutMin=[]  KtOutMax=[]  IntegratorOutMin=[]  IntegratorOutMax=[]  FilterOutMin=[]  FilterOutMax=[]  SumOutMin=[]  SumOutMax=[]  SumI1OutMin=[]  SumI1OutMax=[]  SumI2OutMin=[]  SumI2OutMax=[]  SumI3OutMin=[]  SumI3OutMax=[]  SumDOutMin=[]  SumDOutMax=[]  SaturationOutMin=[]  SaturationOutMax=[]  IntegratorContinuousStateAttributes=''  IntegratorStateMustResolveToSignalObject=off  IntegratorRTWStateStorageClass=Auto  FilterContinuousStateAttributes=''  FilterStateMustResolveToSignalObject=off  FilterRTWStateStorageClass=Auto  DifferentiatorICPrevScaledInput=0  DifferentiatorOutMin=[]  DifferentiatorOutMax=[]  FilterDiffOutCoefMin=[]  FilterDiffOutCoefMax=[]  SumDenOutMin=[]  SumDenOutMax=[]  SumNumOutMin=[]  SumNumOutMax=[]  ReciprocalOutMin=[]  ReciprocalOutMax=[]  DivideOutMin=[]  DivideOutMax=[]  TunerSelectOption=Transfer Function Based (PID Tuner App)
  Solenoids : MATLAB Function  TreatAsAtomicUnit=on
  Sum : Sum  Inputs=|+-
  tag scope: PAM_2_a=global, PAM_2_b=global
  wires:
  Solenoids/3(inside_deadzone_1) -> Delay/1
  Delay/1 -> Solenoids/2(inside_deadzone)
  PID Controller/1 -> Solenoids/1(control)
  Pressure Des/1 -> Sum/1
  [Pressure_2] -> Sum/2
  [deadzone_in] -> Solenoids/3(deadzone_in)
  [deadzone_out] -> Solenoids/4(deadzone_out)
  Solenoids/1(intake) -> [PAM_2_b]
  Solenoids/2(outtake) -> [PAM_2_a]
  [k_i] -> PID Controller/3
  [k_d] -> PID Controller/4
  [N] -> PID Controller/5
  Sum/1 -> PID Controller/1
  [k_p] -> PID Controller/2
  [PAMs_off] -> Solenoids/5(PAMs_on)
  [System_on] -> Solenoids/6(System_on)

== system EPA_Jumper/PAMs/PAM_3 ==
  Pressure Des : Inport
  Delay : Delay  DelayLength=1
  PID Controller : simulink/Continuous/PID Controller  Controller=PID  TimeDomain=Discrete-time  SampleTime=-1  IntegratorMethod=Forward Euler  FilterMethod=Forward Euler  Form=Ideal  UseFilter=on  ControllerParametersSource=external  P=k_p_pam  I=0  D=0.45*0.15/8  N=100  InitialConditionSource=internal  InitialConditionForIntegrator=0  InitialConditionForFilter=0  ExternalReset=none  LimitOutput=off  UpperSaturationLimit=inf  LowerSaturationLimit=-inf  LinearizeAsGain=on  AntiWindupMode=none  Kb=1  TrackingMode=off  Kt=1  PParamMin=[]  PParamMax=[]  IParamMin=[]  IParamMax=[]  DParamMin=[]  DParamMax=[]  NParamMin=[]  NParamMax=[]  KbParamMin=[]  KbParamMax=[]  KtParamMin=[]  KtParamMax=[]  POutMin=[]  POutMax=[]  IOutMin=[]  IOutMax=[]  DOutMin=[]  DOutMax=[]  NOutMin=[]  NOutMax=[]  KbOutMin=[]  KbOutMax=[]  KtOutMin=[]  KtOutMax=[]  IntegratorOutMin=[]  IntegratorOutMax=[]  FilterOutMin=[]  FilterOutMax=[]  SumOutMin=[]  SumOutMax=[]  SumI1OutMin=[]  SumI1OutMax=[]  SumI2OutMin=[]  SumI2OutMax=[]  SumI3OutMin=[]  SumI3OutMax=[]  SumDOutMin=[]  SumDOutMax=[]  SaturationOutMin=[]  SaturationOutMax=[]  IntegratorContinuousStateAttributes=''  IntegratorStateMustResolveToSignalObject=off  IntegratorRTWStateStorageClass=Auto  FilterContinuousStateAttributes=''  FilterStateMustResolveToSignalObject=off  FilterRTWStateStorageClass=Auto  DifferentiatorICPrevScaledInput=0  DifferentiatorOutMin=[]  DifferentiatorOutMax=[]  FilterDiffOutCoefMin=[]  FilterDiffOutCoefMax=[]  SumDenOutMin=[]  SumDenOutMax=[]  SumNumOutMin=[]  SumNumOutMax=[]  ReciprocalOutMin=[]  ReciprocalOutMax=[]  DivideOutMin=[]  DivideOutMax=[]  TunerSelectOption=Transfer Function Based (PID Tuner App)
  Solenoids : MATLAB Function  TreatAsAtomicUnit=on
  Sum : Sum  Inputs=|+-
  tag scope: PAM_3_a=global, PAM_3_b=global
  wires:
  Solenoids/3(inside_deadzone_1) -> Delay/1
  Delay/1 -> Solenoids/2(inside_deadzone)
  Pressure Des/1 -> Sum/1
  [Pressure_3] -> Sum/2
  [deadzone_in] -> Solenoids/3(deadzone_in)
  [deadzone_out] -> Solenoids/4(deadzone_out)
  Solenoids/1(intake) -> [PAM_3_b]
  Solenoids/2(outtake) -> [PAM_3_a]
  [k_i] -> PID Controller/3
  [k_d] -> PID Controller/4
  [N] -> PID Controller/5
  Sum/1 -> PID Controller/1
  PID Controller/1 -> Solenoids/1(control)
  [k_p] -> PID Controller/2
  [PAMs_off] -> Solenoids/5(PAMs_on)
  [System_on] -> Solenoids/6(System_on)

== system EPA_Jumper/PAMs/PAM_4 ==
  Pressure Des : Inport
  Delay : Delay  DelayLength=1
  PID Controller : simulink/Continuous/PID Controller  Controller=PID  TimeDomain=Discrete-time  SampleTime=-1  IntegratorMethod=Forward Euler  FilterMethod=Forward Euler  Form=Ideal  UseFilter=on  ControllerParametersSource=external  P=k_p_pam  I=0  D=0.45*0.15/8  N=100  InitialConditionSource=internal  InitialConditionForIntegrator=0  InitialConditionForFilter=0  ExternalReset=none  LimitOutput=off  UpperSaturationLimit=inf  LowerSaturationLimit=-inf  LinearizeAsGain=on  AntiWindupMode=none  Kb=1  TrackingMode=off  Kt=1  PParamMin=[]  PParamMax=[]  IParamMin=[]  IParamMax=[]  DParamMin=[]  DParamMax=[]  NParamMin=[]  NParamMax=[]  KbParamMin=[]  KbParamMax=[]  KtParamMin=[]  KtParamMax=[]  POutMin=[]  POutMax=[]  IOutMin=[]  IOutMax=[]  DOutMin=[]  DOutMax=[]  NOutMin=[]  NOutMax=[]  KbOutMin=[]  KbOutMax=[]  KtOutMin=[]  KtOutMax=[]  IntegratorOutMin=[]  IntegratorOutMax=[]  FilterOutMin=[]  FilterOutMax=[]  SumOutMin=[]  SumOutMax=[]  SumI1OutMin=[]  SumI1OutMax=[]  SumI2OutMin=[]  SumI2OutMax=[]  SumI3OutMin=[]  SumI3OutMax=[]  SumDOutMin=[]  SumDOutMax=[]  SaturationOutMin=[]  SaturationOutMax=[]  IntegratorContinuousStateAttributes=''  IntegratorStateMustResolveToSignalObject=off  IntegratorRTWStateStorageClass=Auto  FilterContinuousStateAttributes=''  FilterStateMustResolveToSignalObject=off  FilterRTWStateStorageClass=Auto  DifferentiatorICPrevScaledInput=0  DifferentiatorOutMin=[]  DifferentiatorOutMax=[]  FilterDiffOutCoefMin=[]  FilterDiffOutCoefMax=[]  SumDenOutMin=[]  SumDenOutMax=[]  SumNumOutMin=[]  SumNumOutMax=[]  ReciprocalOutMin=[]  ReciprocalOutMax=[]  DivideOutMin=[]  DivideOutMax=[]  TunerSelectOption=Transfer Function Based (PID Tuner App)
  Solenoids : MATLAB Function  TreatAsAtomicUnit=on
  Sum : Sum  Inputs=|+-
  tag scope: PAM_4_a=global, PAM_4_b=global
  wires:
  Solenoids/3(inside_deadzone_1) -> Delay/1
  Delay/1 -> Solenoids/2(inside_deadzone)
  Pressure Des/1 -> Sum/1
  [Pressure_4] -> Sum/2
  [deadzone_in] -> Solenoids/3(deadzone_in)
  [deadzone_out] -> Solenoids/4(deadzone_out)
  Solenoids/1(intake) -> [PAM_4_b]
  Solenoids/2(outtake) -> [PAM_4_a]
  [k_i] -> PID Controller/3
  [k_d] -> PID Controller/4
  [N] -> PID Controller/5
  Sum/1 -> PID Controller/1
  PID Controller/1 -> Solenoids/1(control)
  [k_p] -> PID Controller/2
  [PAMs_off] -> Solenoids/5(PAMs_on)
  [System_on] -> Solenoids/6(System_on)

== system EPA_Jumper/PAMs/PAM_5 ==
  Pressure Des : Inport
  Delay : Delay  DelayLength=1
  PID Controller : simulink/Continuous/PID Controller  Controller=PID  TimeDomain=Discrete-time  SampleTime=-1  IntegratorMethod=Forward Euler  FilterMethod=Forward Euler  Form=Ideal  UseFilter=on  ControllerParametersSource=external  P=k_p_pam  I=0  D=0.45*0.15/8  N=100  InitialConditionSource=internal  InitialConditionForIntegrator=0  InitialConditionForFilter=0  ExternalReset=none  LimitOutput=off  UpperSaturationLimit=inf  LowerSaturationLimit=-inf  LinearizeAsGain=on  AntiWindupMode=none  Kb=1  TrackingMode=off  Kt=1  PParamMin=[]  PParamMax=[]  IParamMin=[]  IParamMax=[]  DParamMin=[]  DParamMax=[]  NParamMin=[]  NParamMax=[]  KbParamMin=[]  KbParamMax=[]  KtParamMin=[]  KtParamMax=[]  POutMin=[]  POutMax=[]  IOutMin=[]  IOutMax=[]  DOutMin=[]  DOutMax=[]  NOutMin=[]  NOutMax=[]  KbOutMin=[]  KbOutMax=[]  KtOutMin=[]  KtOutMax=[]  IntegratorOutMin=[]  IntegratorOutMax=[]  FilterOutMin=[]  FilterOutMax=[]  SumOutMin=[]  SumOutMax=[]  SumI1OutMin=[]  SumI1OutMax=[]  SumI2OutMin=[]  SumI2OutMax=[]  SumI3OutMin=[]  SumI3OutMax=[]  SumDOutMin=[]  SumDOutMax=[]  SaturationOutMin=[]  SaturationOutMax=[]  IntegratorContinuousStateAttributes=''  IntegratorStateMustResolveToSignalObject=off  IntegratorRTWStateStorageClass=Auto  FilterContinuousStateAttributes=''  FilterStateMustResolveToSignalObject=off  FilterRTWStateStorageClass=Auto  DifferentiatorICPrevScaledInput=0  DifferentiatorOutMin=[]  DifferentiatorOutMax=[]  FilterDiffOutCoefMin=[]  FilterDiffOutCoefMax=[]  SumDenOutMin=[]  SumDenOutMax=[]  SumNumOutMin=[]  SumNumOutMax=[]  ReciprocalOutMin=[]  ReciprocalOutMax=[]  DivideOutMin=[]  DivideOutMax=[]  TunerSelectOption=Transfer Function Based (PID Tuner App)
  Solenoids : MATLAB Function  TreatAsAtomicUnit=on
  Sum : Sum  Inputs=|+-
  tag scope: PAM_5_a=global, PAM_5_b=global
  wires:
  Solenoids/3(inside_deadzone_1) -> Delay/1
  Delay/1 -> Solenoids/2(inside_deadzone)
  Pressure Des/1 -> Sum/1
  [Pressure_5] -> Sum/2
  [deadzone_in] -> Solenoids/3(deadzone_in)
  [deadzone_out] -> Solenoids/4(deadzone_out)
  Solenoids/1(intake) -> [PAM_5_b]
  Solenoids/2(outtake) -> [PAM_5_a]
  [k_i] -> PID Controller/3
  [k_d] -> PID Controller/4
  [N] -> PID Controller/5
  Sum/1 -> PID Controller/1
  PID Controller/1 -> Solenoids/1(control)
  [k_p] -> PID Controller/2
  [PAMs_off] -> Solenoids/5(PAMs_on)
  [System_on] -> Solenoids/6(System_on)

== system EPA_Jumper/PAMs/PAM_6 ==
  Pressure Des : Inport
  Delay : Delay  DelayLength=1
  PID Controller : simulink/Continuous/PID Controller  Controller=PID  TimeDomain=Discrete-time  SampleTime=-1  IntegratorMethod=Forward Euler  FilterMethod=Forward Euler  Form=Ideal  UseFilter=on  ControllerParametersSource=external  P=k_p_pam  I=0  D=0.45*0.15/8  N=100  InitialConditionSource=internal  InitialConditionForIntegrator=0  InitialConditionForFilter=0  ExternalReset=none  LimitOutput=off  UpperSaturationLimit=inf  LowerSaturationLimit=-inf  LinearizeAsGain=on  AntiWindupMode=none  Kb=1  TrackingMode=off  Kt=1  PParamMin=[]  PParamMax=[]  IParamMin=[]  IParamMax=[]  DParamMin=[]  DParamMax=[]  NParamMin=[]  NParamMax=[]  KbParamMin=[]  KbParamMax=[]  KtParamMin=[]  KtParamMax=[]  POutMin=[]  POutMax=[]  IOutMin=[]  IOutMax=[]  DOutMin=[]  DOutMax=[]  NOutMin=[]  NOutMax=[]  KbOutMin=[]  KbOutMax=[]  KtOutMin=[]  KtOutMax=[]  IntegratorOutMin=[]  IntegratorOutMax=[]  FilterOutMin=[]  FilterOutMax=[]  SumOutMin=[]  SumOutMax=[]  SumI1OutMin=[]  SumI1OutMax=[]  SumI2OutMin=[]  SumI2OutMax=[]  SumI3OutMin=[]  SumI3OutMax=[]  SumDOutMin=[]  SumDOutMax=[]  SaturationOutMin=[]  SaturationOutMax=[]  IntegratorContinuousStateAttributes=''  IntegratorStateMustResolveToSignalObject=off  IntegratorRTWStateStorageClass=Auto  FilterContinuousStateAttributes=''  FilterStateMustResolveToSignalObject=off  FilterRTWStateStorageClass=Auto  DifferentiatorICPrevScaledInput=0  DifferentiatorOutMin=[]  DifferentiatorOutMax=[]  FilterDiffOutCoefMin=[]  FilterDiffOutCoefMax=[]  SumDenOutMin=[]  SumDenOutMax=[]  SumNumOutMin=[]  SumNumOutMax=[]  ReciprocalOutMin=[]  ReciprocalOutMax=[]  DivideOutMin=[]  DivideOutMax=[]  TunerSelectOption=Transfer Function Based (PID Tuner App)
  Solenoids : MATLAB Function  TreatAsAtomicUnit=on
  Sum : Sum  Inputs=|+-
  tag scope: PAM_6_a=global, PAM_6_b=global
  wires:
  Solenoids/3(inside_deadzone_1) -> Delay/1
  Delay/1 -> Solenoids/2(inside_deadzone)
  Pressure Des/1 -> Sum/1
  [Pressure_6] -> Sum/2
  [deadzone_in] -> Solenoids/3(deadzone_in)
  [deadzone_out] -> Solenoids/4(deadzone_out)
  Solenoids/1(intake) -> [PAM_6_b]
  Solenoids/2(outtake) -> [PAM_6_a]
  [k_i] -> PID Controller/3
  [k_d] -> PID Controller/4
  [N] -> PID Controller/5
  Sum/1 -> PID Controller/1
  PID Controller/1 -> Solenoids/1(control)
  [k_p] -> PID Controller/2
  [PAMs_off] -> Solenoids/5(PAMs_on)
  [System_on] -> Solenoids/6(System_on)

== system EPA_Jumper/PAMs/PAM_7 ==
  Pressure Des : Inport
  Delay : Delay  DelayLength=1
  PID Controller : simulink/Continuous/PID Controller  Controller=PID  TimeDomain=Discrete-time  SampleTime=-1  IntegratorMethod=Forward Euler  FilterMethod=Forward Euler  Form=Ideal  UseFilter=on  ControllerParametersSource=external  P=k_p_pam  I=0  D=0.45*0.15/8  N=100  InitialConditionSource=internal  InitialConditionForIntegrator=0  InitialConditionForFilter=0  ExternalReset=none  LimitOutput=off  UpperSaturationLimit=inf  LowerSaturationLimit=-inf  LinearizeAsGain=on  AntiWindupMode=none  Kb=1  TrackingMode=off  Kt=1  PParamMin=[]  PParamMax=[]  IParamMin=[]  IParamMax=[]  DParamMin=[]  DParamMax=[]  NParamMin=[]  NParamMax=[]  KbParamMin=[]  KbParamMax=[]  KtParamMin=[]  KtParamMax=[]  POutMin=[]  POutMax=[]  IOutMin=[]  IOutMax=[]  DOutMin=[]  DOutMax=[]  NOutMin=[]  NOutMax=[]  KbOutMin=[]  KbOutMax=[]  KtOutMin=[]  KtOutMax=[]  IntegratorOutMin=[]  IntegratorOutMax=[]  FilterOutMin=[]  FilterOutMax=[]  SumOutMin=[]  SumOutMax=[]  SumI1OutMin=[]  SumI1OutMax=[]  SumI2OutMin=[]  SumI2OutMax=[]  SumI3OutMin=[]  SumI3OutMax=[]  SumDOutMin=[]  SumDOutMax=[]  SaturationOutMin=[]  SaturationOutMax=[]  IntegratorContinuousStateAttributes=''  IntegratorStateMustResolveToSignalObject=off  IntegratorRTWStateStorageClass=Auto  FilterContinuousStateAttributes=''  FilterStateMustResolveToSignalObject=off  FilterRTWStateStorageClass=Auto  DifferentiatorICPrevScaledInput=0  DifferentiatorOutMin=[]  DifferentiatorOutMax=[]  FilterDiffOutCoefMin=[]  FilterDiffOutCoefMax=[]  SumDenOutMin=[]  SumDenOutMax=[]  SumNumOutMin=[]  SumNumOutMax=[]  ReciprocalOutMin=[]  ReciprocalOutMax=[]  DivideOutMin=[]  DivideOutMax=[]  TunerSelectOption=Transfer Function Based (PID Tuner App)
  Solenoids : MATLAB Function  TreatAsAtomicUnit=on
  Sum : Sum  Inputs=|+-
  tag scope: PAM_7_a=global, PAM_7_b=global
  wires:
  Solenoids/3(inside_deadzone_1) -> Delay/1
  Delay/1 -> Solenoids/2(inside_deadzone)
  Pressure Des/1 -> Sum/1
  [Pressure_7] -> Sum/2
  [deadzone_in] -> Solenoids/3(deadzone_in)
  [deadzone_out] -> Solenoids/4(deadzone_out)
  Solenoids/1(intake) -> [PAM_7_b]
  Solenoids/2(outtake) -> [PAM_7_a]
  [k_i] -> PID Controller/3
  [k_d] -> PID Controller/4
  [N] -> PID Controller/5
  Sum/1 -> PID Controller/1
  PID Controller/1 -> Solenoids/1(control)
  [k_p] -> PID Controller/2
  [PAMs_off] -> Solenoids/5(PAMs_on)
  [System_on] -> Solenoids/6(System_on)

== system EPA_Jumper/PAMs/PAM_8 ==
  Pressure Des : Inport
  Delay : Delay  DelayLength=1
  PID Controller : simulink/Continuous/PID Controller  Controller=PID  TimeDomain=Discrete-time  SampleTime=-1  IntegratorMethod=Forward Euler  FilterMethod=Forward Euler  Form=Ideal  UseFilter=on  ControllerParametersSource=external  P=k_p_pam  I=0  D=0.45*0.15/8  N=100  InitialConditionSource=internal  InitialConditionForIntegrator=0  InitialConditionForFilter=0  ExternalReset=none  LimitOutput=off  UpperSaturationLimit=inf  LowerSaturationLimit=-inf  LinearizeAsGain=on  AntiWindupMode=none  Kb=1  TrackingMode=off  Kt=1  PParamMin=[]  PParamMax=[]  IParamMin=[]  IParamMax=[]  DParamMin=[]  DParamMax=[]  NParamMin=[]  NParamMax=[]  KbParamMin=[]  KbParamMax=[]  KtParamMin=[]  KtParamMax=[]  POutMin=[]  POutMax=[]  IOutMin=[]  IOutMax=[]  DOutMin=[]  DOutMax=[]  NOutMin=[]  NOutMax=[]  KbOutMin=[]  KbOutMax=[]  KtOutMin=[]  KtOutMax=[]  IntegratorOutMin=[]  IntegratorOutMax=[]  FilterOutMin=[]  FilterOutMax=[]  SumOutMin=[]  SumOutMax=[]  SumI1OutMin=[]  SumI1OutMax=[]  SumI2OutMin=[]  SumI2OutMax=[]  SumI3OutMin=[]  SumI3OutMax=[]  SumDOutMin=[]  SumDOutMax=[]  SaturationOutMin=[]  SaturationOutMax=[]  IntegratorContinuousStateAttributes=''  IntegratorStateMustResolveToSignalObject=off  IntegratorRTWStateStorageClass=Auto  FilterContinuousStateAttributes=''  FilterStateMustResolveToSignalObject=off  FilterRTWStateStorageClass=Auto  DifferentiatorICPrevScaledInput=0  DifferentiatorOutMin=[]  DifferentiatorOutMax=[]  FilterDiffOutCoefMin=[]  FilterDiffOutCoefMax=[]  SumDenOutMin=[]  SumDenOutMax=[]  SumNumOutMin=[]  SumNumOutMax=[]  ReciprocalOutMin=[]  ReciprocalOutMax=[]  DivideOutMin=[]  DivideOutMax=[]  TunerSelectOption=Transfer Function Based (PID Tuner App)
  Solenoids : MATLAB Function  TreatAsAtomicUnit=on
  Sum : Sum  Inputs=|+-
  tag scope: PAM_8_a=global, PAM_8_b=global
  wires:
  Solenoids/3(inside_deadzone_1) -> Delay/1
  Delay/1 -> Solenoids/2(inside_deadzone)
  Pressure Des/1 -> Sum/1
  [Pressure_8] -> Sum/2
  [deadzone_in] -> Solenoids/3(deadzone_in)
  [deadzone_out] -> Solenoids/4(deadzone_out)
  Solenoids/1(intake) -> [PAM_8_b]
  Solenoids/2(outtake) -> [PAM_8_a]
  [k_i] -> PID Controller/3
  [k_d] -> PID Controller/4
  [N] -> PID Controller/5
  Sum/1 -> PID Controller/1
  PID Controller/1 -> Solenoids/1(control)
  [k_p] -> PID Controller/2
  [PAMs_off] -> Solenoids/5(PAMs_on)
  [System_on] -> Solenoids/6(System_on)

== system EPA_Jumper/PAMs/PAM_9 ==
  Pressure Des : Inport
  Delay : Delay  DelayLength=1
  PID Controller : simulink/Continuous/PID Controller  Controller=PID  TimeDomain=Discrete-time  SampleTime=-1  IntegratorMethod=Forward Euler  FilterMethod=Forward Euler  Form=Ideal  UseFilter=on  ControllerParametersSource=external  P=k_p_pam  I=0  D=0.45*0.15/8  N=100  InitialConditionSource=internal  InitialConditionForIntegrator=0  InitialConditionForFilter=0  ExternalReset=none  LimitOutput=off  UpperSaturationLimit=inf  LowerSaturationLimit=-inf  LinearizeAsGain=on  AntiWindupMode=none  Kb=1  TrackingMode=off  Kt=1  PParamMin=[]  PParamMax=[]  IParamMin=[]  IParamMax=[]  DParamMin=[]  DParamMax=[]  NParamMin=[]  NParamMax=[]  KbParamMin=[]  KbParamMax=[]  KtParamMin=[]  KtParamMax=[]  POutMin=[]  POutMax=[]  IOutMin=[]  IOutMax=[]  DOutMin=[]  DOutMax=[]  NOutMin=[]  NOutMax=[]  KbOutMin=[]  KbOutMax=[]  KtOutMin=[]  KtOutMax=[]  IntegratorOutMin=[]  IntegratorOutMax=[]  FilterOutMin=[]  FilterOutMax=[]  SumOutMin=[]  SumOutMax=[]  SumI1OutMin=[]  SumI1OutMax=[]  SumI2OutMin=[]  SumI2OutMax=[]  SumI3OutMin=[]  SumI3OutMax=[]  SumDOutMin=[]  SumDOutMax=[]  SaturationOutMin=[]  SaturationOutMax=[]  IntegratorContinuousStateAttributes=''  IntegratorStateMustResolveToSignalObject=off  IntegratorRTWStateStorageClass=Auto  FilterContinuousStateAttributes=''  FilterStateMustResolveToSignalObject=off  FilterRTWStateStorageClass=Auto  DifferentiatorICPrevScaledInput=0  DifferentiatorOutMin=[]  DifferentiatorOutMax=[]  FilterDiffOutCoefMin=[]  FilterDiffOutCoefMax=[]  SumDenOutMin=[]  SumDenOutMax=[]  SumNumOutMin=[]  SumNumOutMax=[]  ReciprocalOutMin=[]  ReciprocalOutMax=[]  DivideOutMin=[]  DivideOutMax=[]  TunerSelectOption=Transfer Function Based (PID Tuner App)
  Solenoids : MATLAB Function  TreatAsAtomicUnit=on
  Sum : Sum  Inputs=|+-
  tag scope: PAM_9_a=global, PAM_9_b=global
  wires:
  Solenoids/3(inside_deadzone_1) -> Delay/1
  Delay/1 -> Solenoids/2(inside_deadzone)
  Pressure Des/1 -> Sum/1
  [Pressure_9] -> Sum/2
  [deadzone_in] -> Solenoids/3(deadzone_in)
  [deadzone_out] -> Solenoids/4(deadzone_out)
  Solenoids/1(intake) -> [PAM_9_b]
  Solenoids/2(outtake) -> [PAM_9_a]
  [k_i] -> PID Controller/3
  [k_d] -> PID Controller/4
  [N] -> PID Controller/5
  Sum/1 -> PID Controller/1
  PID Controller/1 -> Solenoids/1(control)
  [k_p] -> PID Controller/2
  [PAMs_off] -> Solenoids/5(PAMs_on)
  [System_on] -> Solenoids/6(System_on)

== system EPA_Jumper/Safety /System On ==
  "Simulink Switch " : Inport
  Clock2 : Clock
  Compare To Constant : simulink/Logic and Bit Operations/Compare To Constant  relop=>=  const=10  OutDataTypeStr=boolean
  Data Type Conversion3 : DataTypeConversion  OutDataTypeStr=double
  Emergency Switch : MATLAB Function  TreatAsAtomicUnit=on
  Logical Operator : Logic  Inputs=3  AllPortsSameDT=off  OutDataTypeStr=boolean
  System On : Outport
  Emergency : Outport  Port=2
  wires:
  Emergency Switch/1(y) -> Emergency/1, Logical Operator/3
  [Emergency_Switch] -> Emergency Switch/1(Emergency_switch)
  "Simulink Switch "/1 -> Logical Operator/2
  Clock2/1 -> Compare To Constant/1
  Compare To Constant/1 -> Logical Operator/1
  Logical Operator/1 -> Data Type Conversion3/1
  Data Type Conversion3/1 -> System On/1

== system EPA_Jumper/Ethernet Communication/Inputs/GRF Slave ==
  note: Emergency Switch
  note: GRF
  Data Type Conversion3 : DataTypeConversion
  EtherCAT PDO Receive1 : xpcethercatlib/EtherCAT PDO Receive  Priority=2  sig_name=GRF.Inputs.Byte13  sig_offset=312  sig_type=uint8  type_size=8  sig_dim=1  device_id=0  sample_time=0.001000
      settings: SourceProductName=Simulink Real-Time  SourceProductBaseCode=XP
  "GRFx " : Subsystem
  "GRFy " : Subsystem
  "GRFz " : Subsystem
  tag scope: Emergency_Switch=global
  wires:
  EtherCAT PDO Receive1/1 -> Data Type Conversion3/1
  Data Type Conversion3/1 -> [Emergency_Switch]
